simulink model "s6_template"  (R2023a)
settings: Solver=ode4  StartTime=0.0  StopTime=inf  FixedStep=P_sim_dt  RelTol=1e-3
InitFcn:
  | s6_data;
values from neighbouring files (symbols this model uses):
  CarInputsCmdForward = uint8(1)    [p_mad_car.m]
  P_p_Bf = 0.7    [p_mad_car.m]
  P_p_Br = 0.7    [p_mad_car.m]
  P_p_Cf = 2    [p_mad_car.m]
  P_p_Cr = 2    [p_mad_car.m]
  P_p_delta_max = 21.58/180*pi    (= 0.37664205258)    [p_mad_car.m]
  P_p_Df = 2    [p_mad_car.m]
  P_p_Dr = 2.5    [p_mad_car.m]
  P_p_Ef = -0.1    [p_mad_car.m]
  P_p_Er = -0.05    [p_mad_car.m]
  P_p_J = 192e-6    (= 0.000192)    [p_mad_car.m]
  P_p_k = 2.51    [p_mad_car.m]
  P_p_l = abs(P_p_frontaxle_1 + P_p_rearaxle_1)    [p_mad_car.m]
  P_p_lf = P_p_frontaxle_1    (= 0.05)    [p_mad_car.m]
  P_p_lr = P_p_rearaxle_1    (= 0.049)    [p_mad_car.m]
  P_p_m = 132e-3    (= 0.132)    [p_mad_car.m]
  P_p_T = 316e-3    (= 0.316)    [p_mad_car.m]
  P_p_Tt = P_p_uTt + P_p_output_Tt    (= 0.1)    [p_mad_car.m]
libraries: mad_lib_template x1
settings Model: Creator=hmekiedj  LastModifiedBy=aaron
settings SolverCC: AlgebraicLoopSolver=TrustRegion
settings DataIOCC: ReturnWorkspaceOutputs=off
settings DebuggingCC: SignalInfNanChecking=warning  UnconnectedInputMsg=warning  UnconnectedOutputMsg=warning  UnconnectedLineMsg=warning  ArithmeticOperatorsInVariantConditions=warning
settings ModelReferenceCC: EnableRefExpFcnMdlSchedulingChecks=on
settings SFSimCC: SimUseLocalCustomCode=off  CustomCodeUndefinedFunction=UseInterfaceOnly
settings RTWCC: RTWUseLocalCustomCode=off
settings CodeAppCC: StateflowObjectComments=on

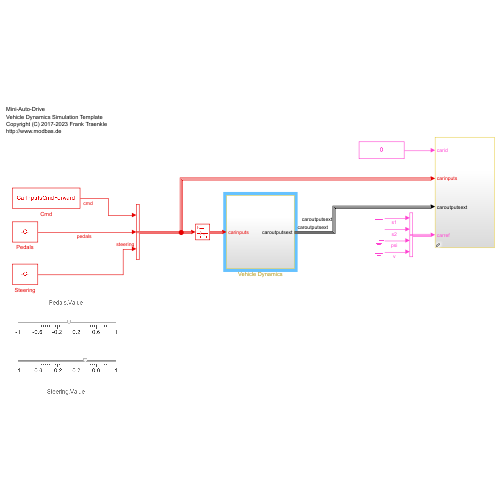
[thumbnail: Simulink's stored preview of the top-level diagram]
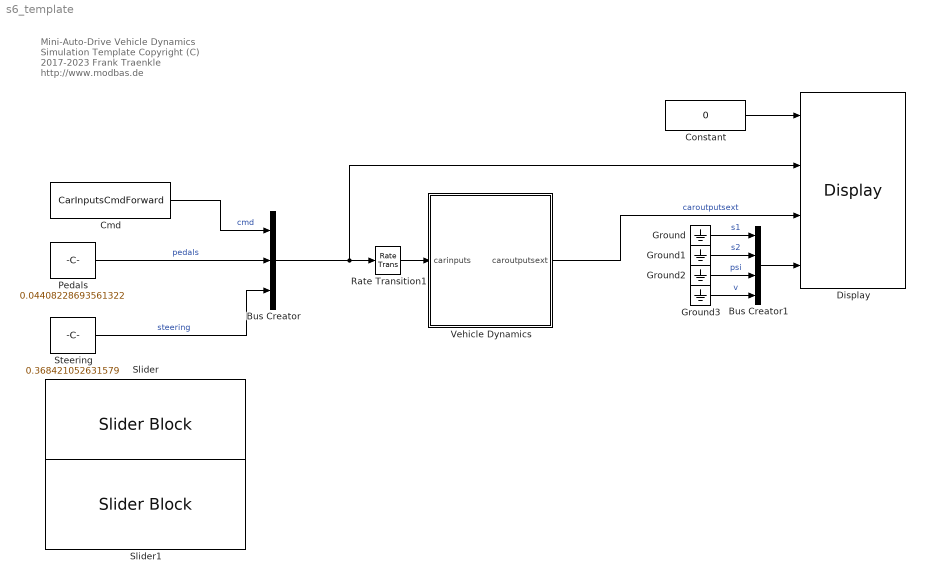
== system s6_template ==
  note: Mini-Auto-Drive
      | Vehicle Dynamics Simulation Template
      | Copyright (C) 2017-2023 Frank Traenkle
      | http://www.modbas.de
  Bus Creator : BusCreator  Inputs=3
  Bus Creator1 : BusCreator  Inputs=4
  Cmd : Constant  Value=CarInputsCmdForward  SampleTime=-1
  Constant : Constant  Value=0
  Display : mad_lib_template/Display  SystemSampleTime=-1  VariantActivationTime=update diagram  Latency=0  AutoFrameSizeCalculation=off
  Ground{,1..3} (4 alike) : Ground
  Pedals : Constant  Value=0.04408228693561322  SampleTime=-1
  Rate Transition1 : RateTransition
  Slider : SliderBlock  ScaleMin=-1  ScaleMax=1
  Slider1 : SliderBlock  LabelPosition=Bottom  ScaleMin=-1  ScaleMax=1
  Steering : Constant  Value=0.368421052631579  SampleTime=-1
  Vehicle Dynamics : Subsystem
  wires:
  Pedals/1 -> Bus Creator/2  "pedals"
  Bus Creator1/1 -> Display/4
  Ground/1 -> Bus Creator1/1  "s1"
  Ground1/1 -> Bus Creator1/2  "s2"
  Ground2/1 -> Bus Creator1/3  "psi"
  Ground3/1 -> Bus Creator1/4  "v"
  Vehicle Dynamics/1(caroutputsext) -> Display/3  "caroutputsext"
  Steering/1 -> Bus Creator/3  "steering"
  Bus Creator/1 -> Display/2, Rate Transition1/1
  Rate Transition1/1 -> Vehicle Dynamics/1(carinputs)
  Constant/1 -> Display/1
  Cmd/1 -> Bus Creator/1  "cmd"

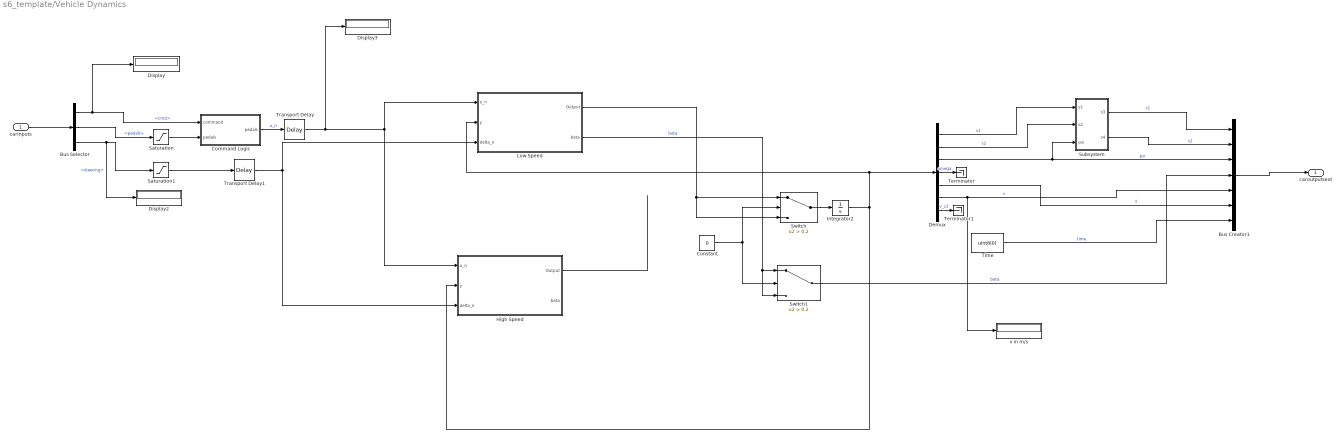
== system s6_template/Vehicle Dynamics ==
  carinputs : Inport
  Bus Creator1 : BusCreator  Inputs=7  OutDataTypeStr=Bus: CAROUTPUTSEXT
  Bus Selector : BusSelector  OutputSignals=cmd,pedals,steering
  Command Logic : MATLAB Function  TreatAsAtomicUnit=on
  Constant : Constant  Value=0
  Demux : Demux  Outputs=7
  Display : Display
  Display2 : Display
  Display3 : Display
  High Speed : Subsystem
  Integrator2 : Integrator
  Low Speed : Subsystem
  Saturation : Saturate  UpperLimit=1  LowerLimit=-1
  Saturation1 : Saturate  UpperLimit=1  LowerLimit=-1
  Subsystem : Subsystem
  Switch : Switch  Criteria=u2 > Threshold  Threshold=0.2  SaturateOnIntegerOverflow=off  InputSameDT=off
  Switch1 : Switch  Criteria=u2 > Threshold  Threshold=0.2  SaturateOnIntegerOverflow=off  InputSameDT=off
  Terminator : Terminator
  Terminator1 : Terminator
  Time : Constant  Value=uint8(0)
  Transport Delay : TransportDelay  DelayTime=P_p_Tt
  Transport Delay1 : TransportDelay  DelayTime=P_p_Tt
  v in m/s : Display
  caroutputsext : Outport  VectorParamsAs1DForOutWhenUnconnected=off
  wires:
  carinputs/1 -> Bus Selector/1
  Bus Selector/2 -> Saturation/1  "<pedals>"
  Bus Selector/3 -> Saturation1/1, Display2/1  "<steering>"
  Demux/3 -> Subsystem/3(psi), Bus Creator1/3  "psi"
  Bus Creator1/1 -> caroutputsext/1
  Demux/6 -> Bus Creator1/5, v in m/s/1  "v"
  Time/1 -> Bus Creator1/7  "time"
  Bus Selector/1 -> Display/1, Command Logic/1(command)  "<cmd>"
  Saturation/1 -> Command Logic/2("pedals ")
  Command Logic/1(pedals) -> Transport Delay/1  "u_n"
  Switch/1 -> Integrator2/1
  Transport Delay/1 -> High Speed/1(u_n), Low Speed/1(u_n), Display3/1
  Saturation1/1 -> Transport Delay1/1
  Low Speed/1(Output) -> Switch/1, Switch/3
  Low Speed/2(beta) -> Switch1/1, Switch1/3  "beta"
  Switch1/1 -> Bus Creator1/4  "beta"
  Demux/4 -> Terminator/1  "omega"
  High Speed/1(Output) -> ?
  Demux/7 -> Terminator1/1  "v_c2"
  Integrator2/1 -> High Speed/2(y), Low Speed/2(y), Demux/1
  Transport Delay1/1 -> High Speed/3(delta_n), Low Speed/3(delta_n)
  Demux/1 -> Subsystem/1(s1)  "s1"
  Demux/2 -> Subsystem/2(s2)  "s2"
  Subsystem/1(s3) -> Bus Creator1/1  "s1"
  Subsystem/2(s4) -> Bus Creator1/2  "s2"
  Constant/1 -> Switch1/2, Switch/2
  Demux/5 -> Bus Creator1/6  "x"

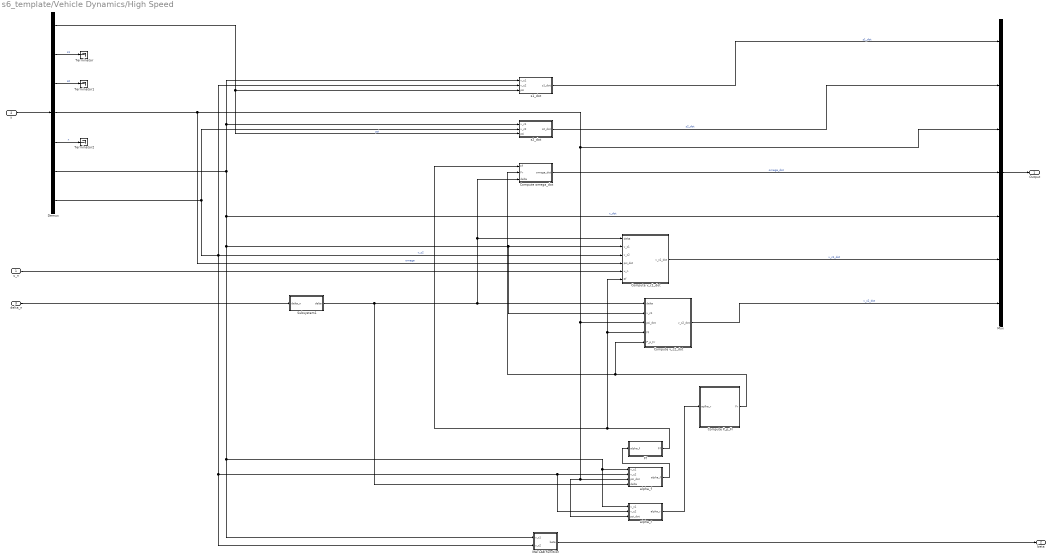
== system s6_template/Vehicle Dynamics/High Speed ==
  u_n : Inport
  y : Inport  Port=2
  delta_n : Inport  Port=3
  Compute P_p_Fr : Subsystem
  Compute omega_dot : Subsystem
  Compute v_c1_dot : Subsystem
  Compute v_c2_dot : Subsystem
  Demux : Demux  Outputs=7
  Ff : Subsystem
  MATLAB Function : MATLAB Function  TreatAsAtomicUnit=on
  Mux : Mux  Inputs=7
  Subsystem1 : Subsystem
  Terminator : Terminator
  Terminator1 : Terminator
  Terminator2 : Terminator
  alpha_f : Subsystem
  alpha_r : Subsystem
  s1_dot : MATLAB Function  TreatAsAtomicUnit=on
  s2_dot : MATLAB Function  TreatAsAtomicUnit=on
  Output : Outport
  beta : Outport  Port=2
  wires:
  Mux/1 -> Output/1
  s1_dot/1(s1_dot) -> Mux/1  "s1_dot"
  Subsystem1/1(delta) -> alpha_f/4(delta), Compute omega_dot/3(delta), Compute v_c1_dot/1(delta), Compute v_c2_dot/1(delta)
  s2_dot/1(s2_dot) -> Mux/2  "s2_dot"
  u_n/1 -> Compute v_c1_dot/5(u_n)
  Demux/2 -> Terminator/1  "s1"
  Demux/3 -> Terminator1/1  "s2"
  Demux/5 -> Terminator2/1  "x"
  Compute v_c1_dot/1(v_c1_dot) -> Mux/6  "v_c1_dot"
  Compute v_c2_dot/1(v_c2_dot) -> Mux/7  "v_c2_dot"
  Demux/7 -> s2_dot/2(v_c2), s1_dot/2(v_c2), Compute v_c1_dot/3(v_c2), alpha_r/2(v_c2), alpha_f/2(v_c2), MATLAB Function/2(v_c2)  "v_c2"
  MATLAB Function/1(beta) -> beta/1
  Compute P_p_Fr/1(Fr) -> Compute omega_dot/2(Fr), Compute v_c2_dot/5(P_p_Fr)
  Ff/1(Ff) -> Compute omega_dot/1(Ff), Compute v_c1_dot/6(Ff), Compute v_c2_dot/4(Ff)
  alpha_f/1(alpha_f) -> Ff/1(alpha_f)
  alpha_r/1(alpha_r) -> Compute P_p_Fr/1(aplha_r)
  delta_n/1 -> Subsystem1/1(delta_n)
  Demux/1 -> s2_dot/3(psi), s1_dot/3(psi)  "psi"
  Demux/4 -> Mux/3, alpha_r/3(psi_dot), alpha_f/3(psi_dot), Compute v_c2_dot/3(psi_dot), Compute v_c1_dot/4(psi_dot)  "omega"
  Compute omega_dot/1(omega_dot) -> Mux/4  "omega_dot"
  y/1 -> Demux/1
  Demux/6 -> Mux/5, alpha_r/1(v_c1), alpha_f/1(v_c1), MATLAB Function/1(v_c1), Compute v_c2_dot/2(v_c1), Compute v_c1_dot/2(v_c1), s2_dot/1(v_c1), s1_dot/1(v_c1)  "x_dot"

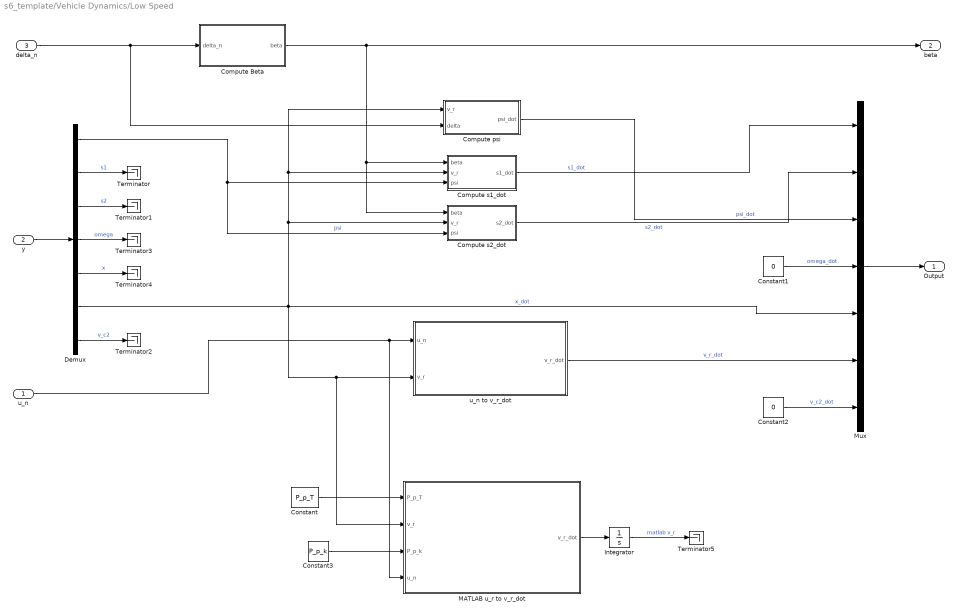
== system s6_template/Vehicle Dynamics/Low Speed ==
  u_n : Inport
  y : Inport  Port=2
  delta_n : Inport  Port=3
  Compute Beta : Subsystem
  Compute psi : Subsystem
  Compute s1_dot : MATLAB Function  TreatAsAtomicUnit=on
  Compute s2_dot : MATLAB Function  TreatAsAtomicUnit=on
  Constant : Constant  Value=P_p_T
  Constant1 : Constant  Value=0
  Constant2 : Constant  Value=0
  Constant3 : Constant  Value=P_p_k
  Demux : Demux  Outputs=7
  Integrator : Integrator
  MATLAB u_r to v_r_dot : MATLAB Function  TreatAsAtomicUnit=on
  Mux : Mux  Inputs=7
  Terminator{,1..5} (6 alike) : Terminator
  u_n to v_r_dot : Subsystem
  Output : Outport
  beta : Outport  Port=2
  wires:
  y/1 -> Demux/1
  Mux/1 -> Output/1
  Demux/1 -> Compute s2_dot/3(psi), Compute s1_dot/3(psi)  "psi"
  delta_n/1 -> Compute psi/2(delta), Compute Beta/1(delta_n)
  Compute s1_dot/1(s1_dot) -> Mux/1  "s1_dot"
  Compute Beta/1(beta) -> Compute s2_dot/1(beta), Compute s1_dot/1(beta), beta/1
  Compute s2_dot/1(s2_dot) -> Mux/2  "s2_dot"
  Compute psi/1(psi_dot) -> Mux/3  "psi_dot"
  Demux/6 -> MATLAB u_r to v_r_dot/2(v_r), u_n to v_r_dot/2(v_r), Mux/5, Compute psi/1(v_r), Compute s1_dot/2(v_r), Compute s2_dot/2(v_r)  "x_dot"
  u_n/1 -> u_n to v_r_dot/1(u_n), MATLAB u_r to v_r_dot/4(u_n)
  Demux/2 -> Terminator/1  "s1"
  Demux/3 -> Terminator1/1  "s2"
  Demux/5 -> Terminator4/1  "x"
  Constant1/1 -> Mux/4  "omega_dot"
  Constant2/1 -> Mux/7  "v_c2_dot"
  Demux/4 -> Terminator3/1  "omega"
  Demux/7 -> Terminator2/1  "v_c2"
  Constant/1 -> MATLAB u_r to v_r_dot/1(P_p_T)
  Constant3/1 -> MATLAB u_r to v_r_dot/3(P_p_k)
  MATLAB u_r to v_r_dot/1(v_r_dot) -> Integrator/1
  u_n to v_r_dot/1(v_r_dot) -> Mux/6  "v_r_dot"
  Integrator/1 -> Terminator5/1  "matlab v_r"

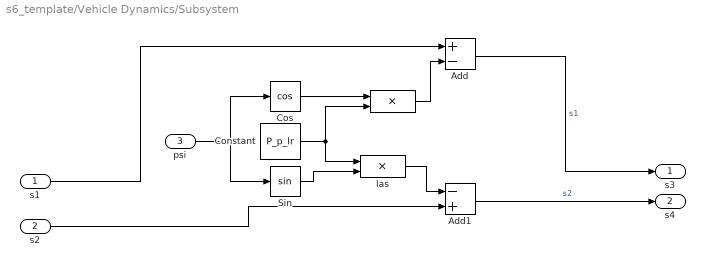
== system s6_template/Vehicle Dynamics/Subsystem ==
  s1 : Inport
  s2 : Inport  Port=2
  psi : Inport  Port=3
  " " : Product
  Add : Sum  Inputs=+-
  Add1 : Sum  Inputs=-+
  Constant : Constant  Value=P_p_lr
  Cos : Trigonometry  Operator=cos
  Sin : Trigonometry
  las : Product
  s3 : Outport
  s4 : Outport  Port=2
  wires:
  Constant/1 -> " "/2, las/1
  Cos/1 -> " "/1
  " "/1 -> Add/2
  psi/1 -> Sin/1, Cos/1
  Sin/1 -> las/2
  las/1 -> Add1/1
  s1/1 -> Add/1
  Add/1 -> s3/1  "s1"
  Add1/1 -> s4/1  "s2"
  s2/1 -> Add1/2

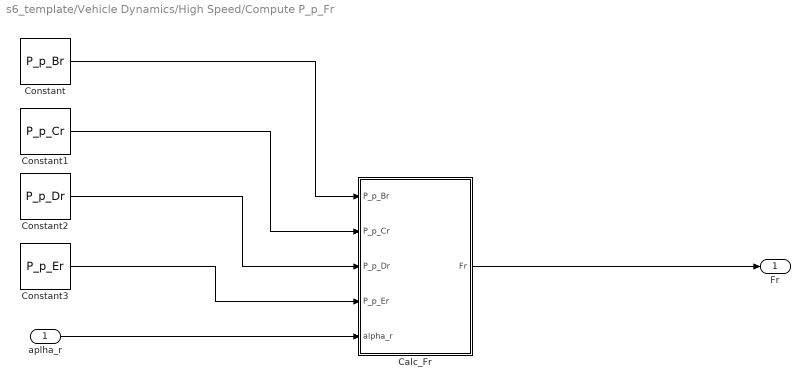
== system s6_template/Vehicle Dynamics/High Speed/Compute P_p_Fr ==
  aplha_r : Inport
  Calc_Fr : MATLAB Function  TreatAsAtomicUnit=on
  Constant : Constant  Value=P_p_Br
  Constant1 : Constant  Value=P_p_Cr
  Constant2 : Constant  Value=P_p_Dr
  Constant3 : Constant  Value=P_p_Er
  Fr : Outport
  wires:
  aplha_r/1 -> Calc_Fr/5(alpha_r)
  Constant3/1 -> Calc_Fr/4(P_p_Er)
  Constant2/1 -> Calc_Fr/3(P_p_Dr)
  Constant1/1 -> Calc_Fr/2(P_p_Cr)
  Constant/1 -> Calc_Fr/1(P_p_Br)
  Calc_Fr/1(Fr) -> Fr/1

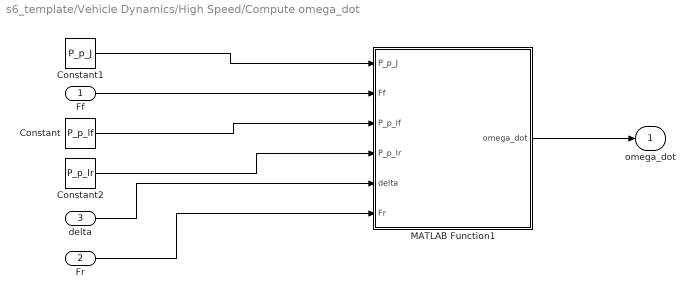
== system s6_template/Vehicle Dynamics/High Speed/Compute omega_dot ==
  Ff : Inport
  Fr : Inport  Port=2
  delta : Inport  Port=3
  Constant : Constant  Value=P_p_lf
  Constant1 : Constant  Value=P_p_J
  Constant2 : Constant  Value=P_p_lr
  MATLAB Function1 : MATLAB Function  TreatAsAtomicUnit=on
  omega_dot : Outport
  wires:
  MATLAB Function1/1(omega_dot) -> omega_dot/1
  Constant1/1 -> MATLAB Function1/1(P_p_J)
  Ff/1 -> MATLAB Function1/2(Ff)
  Fr/1 -> MATLAB Function1/6(Fr)
  Constant/1 -> MATLAB Function1/3(P_p_lf)
  Constant2/1 -> MATLAB Function1/4(P_p_lr)
  delta/1 -> MATLAB Function1/5(delta)

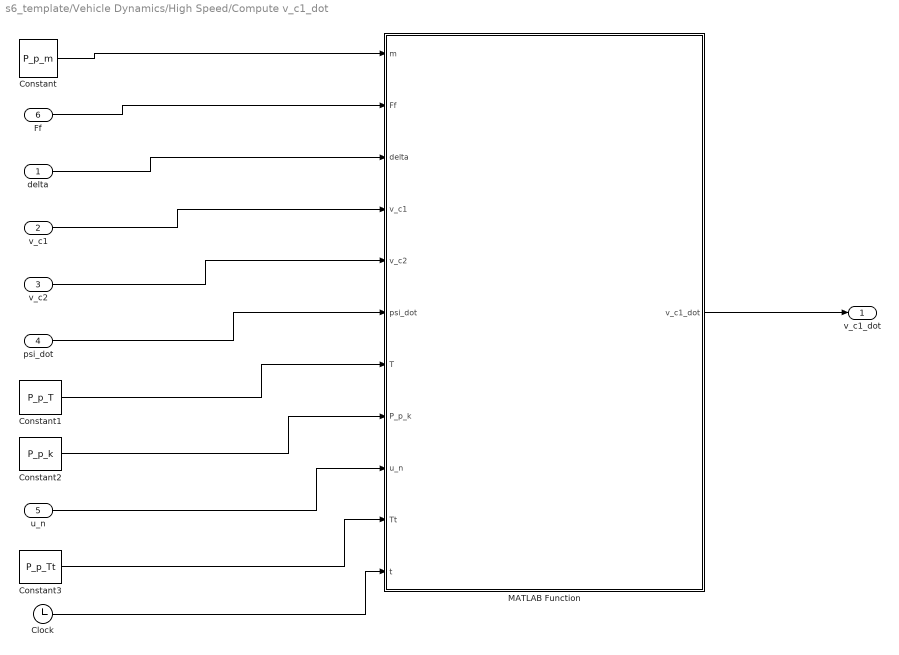
== system s6_template/Vehicle Dynamics/High Speed/Compute v_c1_dot ==
  delta : Inport
  v_c1 : Inport  Port=2
  v_c2 : Inport  Port=3
  psi_dot : Inport  Port=4
  u_n : Inport  Port=5
  Ff : Inport  Port=6
  Clock : Clock
  Constant : Constant  Value=P_p_m
  Constant1 : Constant  Value=P_p_T
  Constant2 : Constant  Value=P_p_k
  Constant3 : Constant  Value=P_p_Tt
  MATLAB Function : MATLAB Function  TreatAsAtomicUnit=on
  v_c1_dot : Outport
  wires:
  MATLAB Function/1(v_c1_dot) -> v_c1_dot/1
  delta/1 -> MATLAB Function/3(delta)
  v_c1/1 -> MATLAB Function/4(v_c1)
  v_c2/1 -> MATLAB Function/5(v_c2)
  psi_dot/1 -> MATLAB Function/6(psi_dot)
  u_n/1 -> MATLAB Function/9(u_n)
  Constant/1 -> MATLAB Function/1(m)
  Ff/1 -> MATLAB Function/2(Ff)
  Constant1/1 -> MATLAB Function/7(T)
  Constant2/1 -> MATLAB Function/8(P_p_k)
  Constant3/1 -> MATLAB Function/10(Tt)
  Clock/1 -> MATLAB Function/11(t)

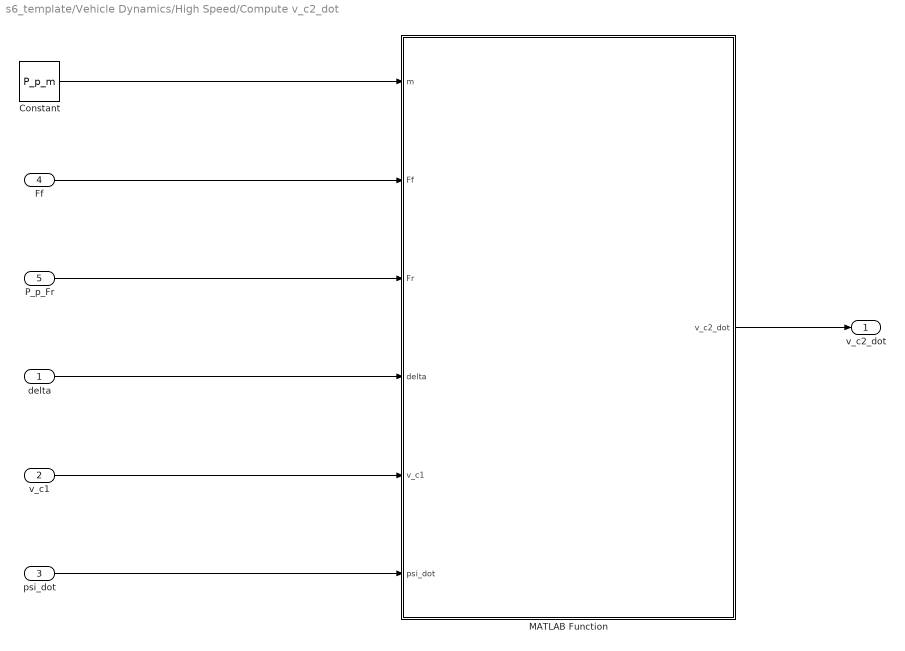
== system s6_template/Vehicle Dynamics/High Speed/Compute v_c2_dot ==
  delta : Inport
  v_c1 : Inport  Port=2
  psi_dot : Inport  Port=3
  Ff : Inport  Port=4
  P_p_Fr : Inport  Port=5
  Constant : Constant  Value=P_p_m
  MATLAB Function : MATLAB Function  TreatAsAtomicUnit=on
  v_c2_dot : Outport
  wires:
  MATLAB Function/1(v_c2_dot) -> v_c2_dot/1
  delta/1 -> MATLAB Function/4(delta)
  v_c1/1 -> MATLAB Function/5(v_c1)
  P_p_Fr/1 -> MATLAB Function/3(Fr)
  psi_dot/1 -> MATLAB Function/6(psi_dot)
  Constant/1 -> MATLAB Function/1(m)
  Ff/1 -> MATLAB Function/2(Ff)

== system s6_template/Vehicle Dynamics/High Speed/Ff ==
  alpha_f : Inport
  Calc_Ff : MATLAB Function  TreatAsAtomicUnit=on
  Constant : Constant  Value=P_p_Bf
  Constant1 : Constant  Value=P_p_Cf
  Constant2 : Constant  Value=P_p_Df
  Constant3 : Constant  Value=P_p_Ef
  Ff : Outport
  wires:
  alpha_f/1 -> Calc_Ff/5(alpha_f)
  Constant1/1 -> Calc_Ff/2(P_p_Cf)
  Constant/1 -> Calc_Ff/1(P_p_Bf)
  Constant3/1 -> Calc_Ff/4(P_p_Ef)
  Constant2/1 -> Calc_Ff/3(P_p_Df)
  Calc_Ff/1(Ff) -> Ff/1

== system s6_template/Vehicle Dynamics/High Speed/Subsystem1 ==
  delta_n : Inport
  Clock : Clock
  Constant : Constant  Value=P_p_delta_max
  Constant1 : Constant  Value=P_p_Tt
  MATLAB Function : MATLAB Function  TreatAsAtomicUnit=on
  delta : Outport
  wires:
  MATLAB Function/1(delta) -> delta/1
  Clock/1 -> MATLAB Function/3(t)
  Constant1/1 -> MATLAB Function/4(P_p_Tt)
  Constant/1 -> MATLAB Function/2(delta_n)
  delta_n/1 -> MATLAB Function/1(P_p_delta_max)

== system s6_template/Vehicle Dynamics/High Speed/alpha_f ==
  v_c1 : Inport
  v_c2 : Inport  Port=2
  psi_dot : Inport  Port=3
  delta : Inport  Port=4
  Constant : Constant  Value=P_p_lf
  MATLAB Function : MATLAB Function  TreatAsAtomicUnit=on
  alpha_f : Outport
  wires:
  v_c1/1 -> MATLAB Function/1(v_c1)
  v_c2/1 -> MATLAB Function/2(v_c2)
  Constant/1 -> MATLAB Function/3(P_p_lf)
  psi_dot/1 -> MATLAB Function/4(psi_dot)
  MATLAB Function/1(alpha_f) -> alpha_f/1
  delta/1 -> MATLAB Function/5(delta)

== system s6_template/Vehicle Dynamics/High Speed/alpha_r ==
  v_c1 : Inport
  v_c2 : Inport  Port=2
  psi_dot : Inport  Port=3
  Constant : Constant  Value=P_p_lr
  MATLAB Function : MATLAB Function  TreatAsAtomicUnit=on
  alpha_r : Outport
  wires:
  v_c1/1 -> MATLAB Function/1(v_c1)
  v_c2/1 -> MATLAB Function/2(v_c2)
  Constant/1 -> MATLAB Function/3(P_p_lr)
  psi_dot/1 -> MATLAB Function/4(psi_dot)
  MATLAB Function/1(alpha_r) -> alpha_r/1

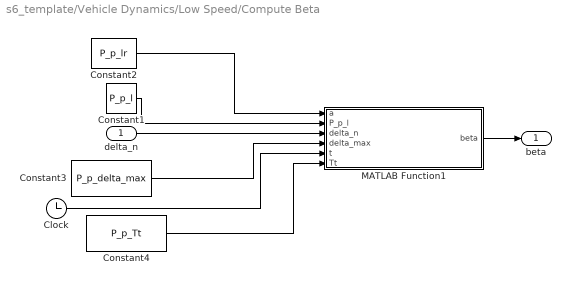
== system s6_template/Vehicle Dynamics/Low Speed/Compute Beta ==
  delta_n : Inport
  Clock : Clock
  Constant1 : Constant  Value=P_p_l
  Constant2 : Constant  Value=P_p_lr
  Constant3 : Constant  Value=P_p_delta_max
  Constant4 : Constant  Value=P_p_Tt
  MATLAB Function1 : MATLAB Function  TreatAsAtomicUnit=on
  beta : Outport
  wires:
  Constant3/1 -> MATLAB Function1/4(delta_max)
  Constant1/1 -> MATLAB Function1/2(P_p_l)
  Constant4/1 -> MATLAB Function1/6(Tt)
  MATLAB Function1/1(beta) -> beta/1
  Constant2/1 -> MATLAB Function1/1(a)
  Clock/1 -> MATLAB Function1/5(t)
  delta_n/1 -> MATLAB Function1/3(delta_n)

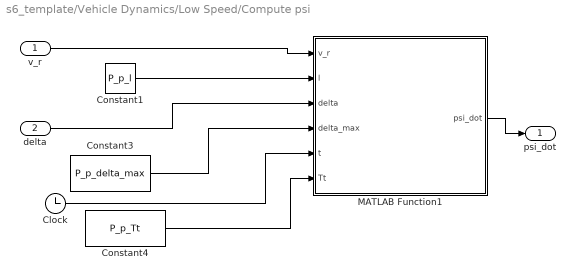
== system s6_template/Vehicle Dynamics/Low Speed/Compute psi ==
  v_r : Inport
  delta : Inport  Port=2
  Clock : Clock
  Constant1 : Constant  Value=P_p_l
  Constant3 : Constant  Value=P_p_delta_max
  Constant4 : Constant  Value=P_p_Tt
  MATLAB Function1 : MATLAB Function  TreatAsAtomicUnit=on
  psi_dot : Outport
  wires:
  Constant3/1 -> MATLAB Function1/4(delta_max)
  Constant1/1 -> MATLAB Function1/2(l)
  Constant4/1 -> MATLAB Function1/6(Tt)
  MATLAB Function1/1(psi_dot) -> psi_dot/1
  v_r/1 -> MATLAB Function1/1(v_r)
  Clock/1 -> MATLAB Function1/5(t)
  delta/1 -> MATLAB Function1/3(delta)

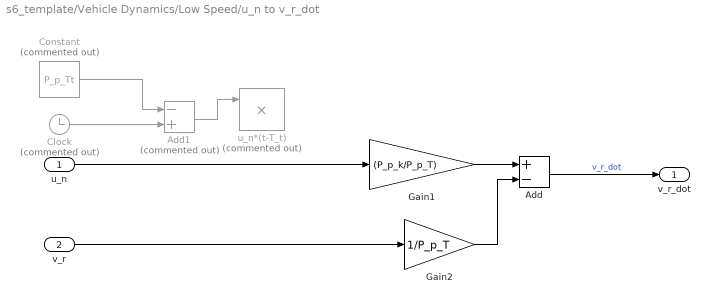
== system s6_template/Vehicle Dynamics/Low Speed/u_n to v_r_dot ==
  u_n : Inport
  v_r : Inport  Port=2
  Add : Sum  Inputs=+-
  Add1 : Sum  Commented=on  Inputs=-+
  Clock : Clock  Commented=on
  Constant : Constant  Commented=on  Value=P_p_Tt
  Gain1 : Gain  Gain=(P_p_k/P_p_T)
  Gain2 : Gain  Gain=1/P_p_T
  u_n*(t-T_t) : Product  Commented=on
  v_r_dot : Outport
  wires:
  Gain2/1 -> Add/2
  Clock/1 -> Add1/2
  u_n/1 -> Gain1/1
  Add1/1 -> u_n*(t-T_t)/1
  Constant/1 -> Add1/1
  Gain1/1 -> Add/1
  Add/1 -> v_r_dot/1  "v_r_dot"
  v_r/1 -> Gain2/1

== matlab function s6_template/Vehicle Dynamics/Low Speed/Compute psi/MATLAB Function1 ==
  data: v_r input; psi_dot output; l input; delta input; delta_max input; t input; Tt input
function psi_dot = fcn(v_r, l, delta, delta_max, t, Tt)

% psi = (v_r/l) * tan(delta_max * delta * (t - Tt) );
psi_dot = (v_r/l) * tan(delta_max * delta);

== matlab function s6_template/Vehicle Dynamics/High Speed/Compute v_c1_dot/MATLAB Function ==
  data: m input; v_c1_dot output; Ff input; delta input; v_c1 input; v_c2 input; psi_dot input; T input; P_p_k input; u_n input; Tt input; t input
function v_c1_dot = fcn(m, Ff, delta, v_c1, v_c2, psi_dot, T, P_p_k, u_n, Tt, t)

% v_c1_dot = (1/m) * (-Ff * sin(delta) + m * v_c2 * psi_dot) ...
%                     - 1/T * v_c1 ...
%                     + (P_p_k/T) * u_n * (t - Tt);


v_c1_dot = (1/m) * (-Ff * sin(delta) + m * v_c2 * psi_dot) ...
                    - 1/T * v_c1 ...
                    + (P_p_k/T) * u_n;

== matlab function s6_template/Vehicle Dynamics/High Speed/Compute v_c2_dot/MATLAB Function ==
  data: m input; v_c2_dot output; Ff input; Fr input; delta input; v_c1 input; psi_dot input
function v_c2_dot = fcn(m, Ff, Fr, delta, v_c1, psi_dot)

v_c2_dot = (1/m) * (Ff * cos(delta) + Fr - m * v_c1 * psi_dot);

== matlab function s6_template/Vehicle Dynamics/High Speed/Compute P_p_Fr/Calc_Fr ==
  data: P_p_Br input; Fr output; P_p_Cr input; P_p_Dr input; P_p_Er input; alpha_r input
function Fr = fcn(P_p_Br, P_p_Cr, P_p_Dr, P_p_Er, alpha_r)

Fr = P_p_Dr * sin(P_p_Cr * atan(P_p_Br * (1 - P_p_Er) * alpha_r ...
    - P_p_Er * atan(P_p_Br * alpha_r)));

== matlab function s6_template/Vehicle Dynamics/High Speed/Ff/Calc_Ff ==
  data: P_p_Bf input; Ff output; P_p_Cf input; P_p_Df input; P_p_Ef input; alpha_f input
function Ff = fcn(P_p_Bf, P_p_Cf, P_p_Df, P_p_Ef, alpha_f)

Ff = P_p_Df * sin(P_p_Cf * atan(P_p_Bf * (1 - P_p_Ef) * alpha_f ...
    - P_p_Ef * atan(P_p_Bf * alpha_f)));

== matlab function s6_template/Vehicle Dynamics/High Speed/alpha_r/MATLAB Function ==
  data: v_c1 input; alpha_r output; v_c2 input; P_p_lr input; psi_dot input
function alpha_r = fcn(v_c1, v_c2, P_p_lr, psi_dot)

if(v_c1 > 0)
    % we will use this equvaltion if the vilocity v_c1 is above 0 (v_c1 > 0)
    alpha_r = -atan((v_c2 - P_p_lr * psi_dot) / v_c1);
elseif (v_c1 < 0)
    % we will use this equvaltion if the vilocity v_c1 is below 0 (v_c1 < 0)
    alpha_r = atan((v_c2 - P_p_lr * psi_dot) / v_c1);
else
    alpha_r = 0;
end

== matlab function s6_template/Vehicle Dynamics/Low Speed/MATLAB u_r to v_r_dot ==
  data: P_p_T input; v_r_dot output; v_r input; P_p_k input; u_n input
function v_r_dot = fcn(P_p_T, v_r, P_p_k, u_n)

v_r_dot = (-1/P_p_T) * v_r + (P_p_k/P_p_T) * u_n;

== matlab function s6_template/Vehicle Dynamics/High Speed/Subsystem1/MATLAB Function ==
  data: P_p_delta_max input; delta output; delta_n input; t input; P_p_Tt input
function delta = fcn(P_p_delta_max, delta_n, t, P_p_Tt)

% delta = P_p_delta_max * delta_n*(t-P_p_Tt);
delta = P_p_delta_max * delta_n;

== matlab function s6_template/Vehicle Dynamics/High Speed/alpha_f/MATLAB Function ==
  data: v_c1 input; alpha_f output; v_c2 input; P_p_lf input; psi_dot input; delta input
function alpha_f = fcn(v_c1, v_c2, P_p_lf, psi_dot, delta)

if (v_c1 > 0)
    % we will use this equvaltion if the vilocity v_c1 is above 0 (v_c1 > 0)
    alpha_f = -atan((v_c2 + P_p_lf * psi_dot) / v_c1) + delta;
elseif (v_c1 < 0)
    % we will use this equvaltion if the vilocity v_c1 is below 0 (v_c1 < 0)
    alpha_f = atan((v_c2 + P_p_lf * psi_dot) / v_c1) - delta;
else
    alpha_f = 0;
end

== matlab function s6_template/Vehicle Dynamics/Command Logic ==
  data: command input; pedals input; pedals output
function pedals = fcn(command, pedals)
    switch command
        case 0      % CarInputsCmdHalt
            pedals = 0;
        case 1  % CarInputsCmdForward 
            if (pedals < 0)
                pedals = 0;
            end
        case 2  % CarInputsCmdReverse 
            if (pedals > 0)
                pedals = 0;
            end
     end
end

== matlab function s6_template/Vehicle Dynamics/High Speed/MATLAB Function ==
  data: v_c1 input; beta output; v_c2 input
function beta = fcn(v_c1, v_c2)

beta = atan2(v_c2, v_c1);

== matlab function s6_template/Vehicle Dynamics/High Speed/Compute omega_dot/MATLAB Function1 ==
  data: P_p_J input; omega_dot output; Ff input; P_p_lf input; P_p_lr input; delta input; Fr input
function omega_dot = fcn(P_p_J, Ff, P_p_lf, P_p_lr, delta, Fr)

omega_dot = (1/P_p_J) * (Ff * P_p_lf * cos(delta) - Fr * P_p_lr);

== matlab function s6_template/Vehicle Dynamics/Low Speed/Compute Beta/MATLAB Function1 ==
  data: a input; beta output; P_p_l input; delta_n input; delta_max input; t input; Tt input
function beta = fcn(a, P_p_l, delta_n, delta_max, t, Tt)

% beta = atan((a/l) * tan(delta_max*delta_n*(t - Tt) )  );
beta = atan( (a/P_p_l) * tan(delta_max * delta_n)  );

== matlab function s6_template/Vehicle Dynamics/High Speed/s2_dot ==
  data: v_c1 input; v_c2 input; s2_dot output; psi input
function s2_dot = fcn(v_c1, v_c2, psi)

s2_dot = v_c1 * sin(psi) + v_c2 * cos(psi);

== matlab function s6_template/Vehicle Dynamics/High Speed/s1_dot ==
  data: v_c1 input; v_c2 input; s1_dot output; psi input
function s1_dot = fcn(v_c1, v_c2, psi)

s1_dot = v_c1 * cos(psi) - v_c2 * sin(psi);

== matlab function s6_template/Vehicle Dynamics/Low Speed/Compute s2_dot ==
  data: beta input; v_r input; s2_dot output; psi input
function s2_dot = fcn(beta, v_r, psi)

s2_dot = (v_r/cos(beta)) * sin(psi + beta);

== matlab function s6_template/Vehicle Dynamics/Low Speed/Compute s1_dot ==
  data: beta input; v_r input; s1_dot output; psi input
function s1_dot = fcn(beta,v_r, psi)

s1_dot =  (v_r/cos(beta))  * cos(psi + beta);
